simulink model "SegwayV2"  (R2021a)
settings: Solver=VariableStepAuto  StartTime=0.0  StopTime=15  RelTol=1e-3
values from neighbouring files (symbols this model uses):
  B = [0 ; B2 ; 0 ; B4;]    [Segway_modelV1.m]    (also in Segway_modelV2.m)
  C = [1 0 0 0 ... (first row only)    [Segway_modelV1.m]    (also in Segway_modelV2.m)
  X0 = [0 ;0 ;0 ;0;]    [Segway_modelV1.m]    (also in Segway_modelV2.m)
undefined symbols (not defined in the file or in its folder): K
settings Model: Creator=Akshit  LastModifiedBy=mluser
settings SolverCC: AlgebraicLoopSolver=TrustRegion
settings DebuggingCC: SFMachineParentedDataDiag=warning

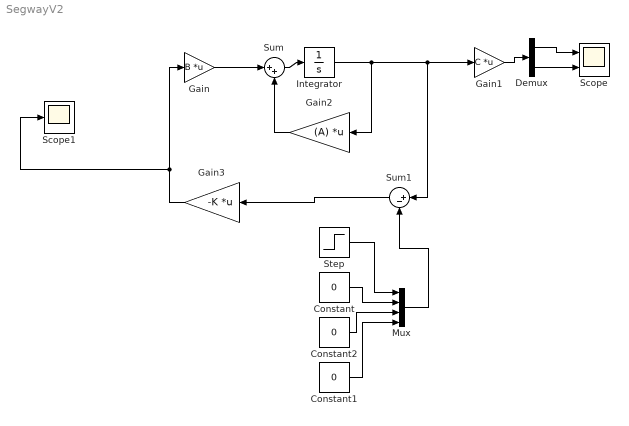
== system SegwayV2 ==
  Constant : Constant  Value=0
  Constant1 : Constant  Value=0
  Constant2 : Constant  Value=0
  Demux : Demux  Outputs=2
  Gain : Gain  Gain=B  Multiplication=Matrix(K*u)
  Gain1 : Gain  Gain=C  Multiplication=Matrix(K*u)
  Gain2 : Gain  Gain=(A)  Multiplication=Matrix(K*u)
  Gain3 : Gain  Gain=-K  Multiplication=Matrix(K*u)
  Integrator : Integrator  InitialCondition=X0
  Mux : Mux
  Scope : Scope  NumInputPorts=2
  Scope1 : Scope
  Step : Step  Time=0  SampleTime=0
  Sum : Sum  Inputs=|++
  Sum1 : Sum  Inputs=|+-
  wires:
  Gain/1 -> Sum/1
  Sum/1 -> Integrator/1
  Integrator/1 -> Gain2/1, Sum1/1, Gain1/1
  Gain2/1 -> Sum/2
  Gain1/1 -> Demux/1
  Demux/1 -> Scope/1
  Demux/2 -> Scope/2
  Gain3/1 -> Scope1/1, Gain/1
  Sum1/1 -> Gain3/1
  Mux/1 -> Sum1/2
  Step/1 -> Mux/1
  Constant/1 -> Mux/2
  Constant1/1 -> Mux/4
  Constant2/1 -> Mux/3
